simulink model "MBD_W2_P4"  (R2020a)
settings: Solver=ode15s  StartTime=0.0  StopTime=0.2  RelTol=1e-3
values from neighbouring files (symbols this model uses):
  b = 3.5077E-6    [MBD_W2_P4_DataDictionary.sldd]    (also in MBD_W2_P4_Workspace.mat = 3.5077e-06)
  J = 3.2284E-6    [MBD_W2_P4_DataDictionary.sldd]    (also in MBD_W2_P4_Workspace.mat = 3.2284e-06)
  Ke = 0.0274    [MBD_W2_P4_DataDictionary.sldd]    (also in MBD_W2_P4_Workspace.mat)
  Kt = 0.0274    [MBD_W2_P4_DataDictionary.sldd]    (also in MBD_W2_P4_Workspace.mat)
  L = 2.75E-6    [MBD_W2_P4_DataDictionary.sldd]    (also in MBD_W2_P4_Workspace.mat = 2.75e-06)
  R = 4.0    [MBD_W2_P4_DataDictionary.sldd]    (also in MBD_W2_P4_Workspace.mat = 4)
settings Model: Creator=Atri Mondal  LastModifiedBy=Atri Mondal

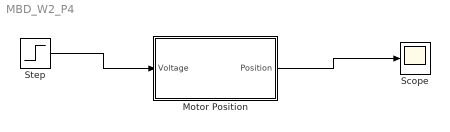
== system MBD_W2_P4 ==
  Motor Position : Subsystem
  Scope : Scope
  Step : Step  Time=0  SampleTime=0
  wires:
  Step/1 -> Motor Position/1(Voltage)
  Motor Position/1(Position) -> Scope/1

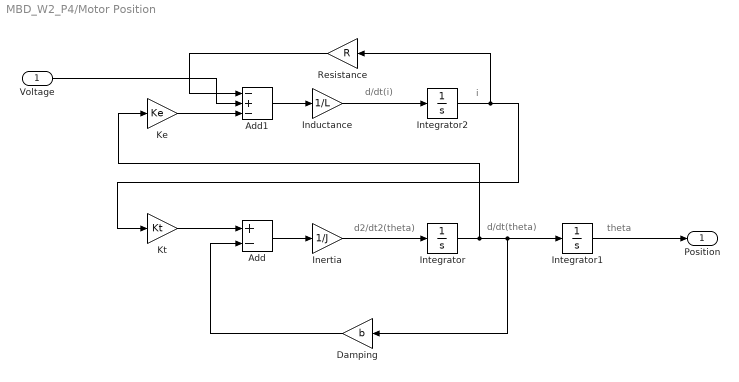
== system MBD_W2_P4/Motor Position ==
  note: d/dt(i)
  note: d2/dt2(theta)
  note: i
  note: d/dt(theta)
  note: theta
  Voltage : Inport
  Add : Sum  Inputs=+-
  Add1 : Sum  Inputs=-+-
  Damping : Gain  Gain=b
  Inductance : Gain  Gain=1/L
  Inertia : Gain  Gain=1/J
  Integrator : Integrator
  Integrator1 : Integrator
  Integrator2 : Integrator
  Ke : Gain  Gain=Ke
  Kt : Gain  Gain=Kt
  Resistance : Gain  Gain=R
  Position : Outport
  wires:
  Ke/1 -> Add1/3
  Add/1 -> Inertia/1
  Integrator/1 -> Ke/1, Damping/1, Integrator1/1
  Voltage/1 -> Add1/2
  Kt/1 -> Add/1
  Integrator2/1 -> Resistance/1, Kt/1
  Damping/1 -> Add/2
  Integrator1/1 -> Position/1
  Add1/1 -> Inductance/1
  Inertia/1 -> Integrator/1
  Resistance/1 -> Add1/1
  Inductance/1 -> Integrator2/1
